simulink model "pv_model"  (R2020a)
settings: Solver=VariableStepAuto  StartTime=0.0  StopTime=4  RelTol=1e-3
undefined symbols (not defined in the file): Eg0, Isc, K, Ki, n, Ns, q, Rs, Rsh, Tn, Voc
libraries: simulink x3
settings Model: Creator=vardh  LastModifiedBy=vardh
settings SolverCC: AlgebraicLoopSolver=LineSearch
settings DebuggingCC: AlgebraicLoopMsg=none

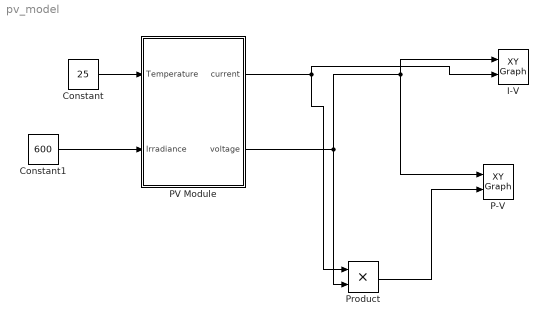
== system pv_model ==
  Constant : Constant  Value=25
  Constant1 : Constant  Value=600
  "I-V " : simulink/Sinks/XY Graph  xmin=0  xmax=35  ymin=0  ymax=10  st=-1
  P-V : simulink/Sinks/XY Graph  xmin=0  xmax=35  ymin=0  ymax=210  st=-1
  PV Module : Subsystem  InitFcn=|
      | Ki=0.0032;
      | q=1.6e-19;
      | K=1.38e-23;
      | n=1.3;
      | Eg0=1.1;
      | Rs=0.221;
      | Rsh=415.405;
      | Tn=298;
      | Voc=32.9;
      | Isc=8.21;
      | Ns=54;
  Product : Product
  wires:
  Constant/1 -> PV Module/1(Temperature)
  Constant1/1 -> PV Module/2(Irradiance)
  PV Module/1(current) -> Product/1, "I-V "/2
  PV Module/2(voltage) -> P-V/1, "I-V "/1, Product/2
  Product/1 -> P-V/2

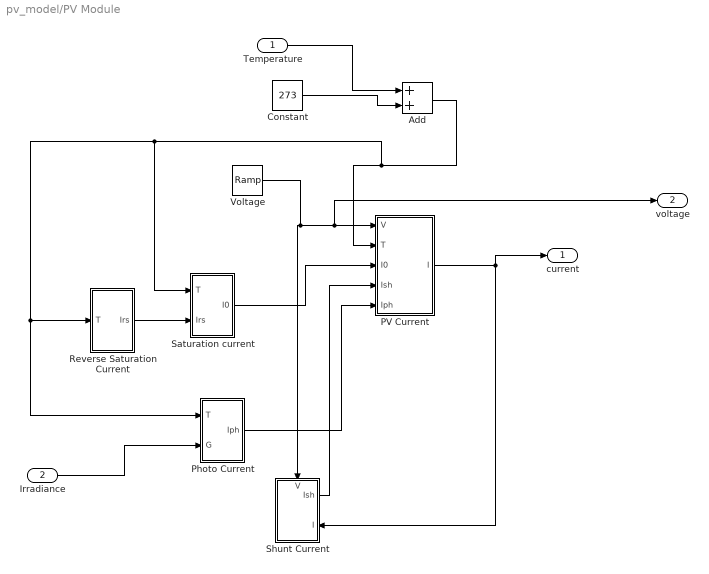
== system pv_model/PV Module ==
  Temperature : Inport
  Irradiance : Inport  Port=2
  Add : Sum
  Constant : Constant  Value=273
  PV Current : Subsystem
  Photo Current : Subsystem
  Reverse Saturation Current : Subsystem
  Saturation current : Subsystem
  Shunt Current : Subsystem
      settings: PortSchema="{\"entries\":[{\"content\":{\"sides\":[{\"content\":{\"connectorIds\":[]},\"type\":\"ConnectorPlacement.EquallySpacedRectSide\",\"uuid\":\"dfbb4c5d-8fcf-4819-9965-5f47220c7753\"},{\"content\":{\"connectorIds\":[\"Out1\",\"In2\"],\"side\":\"RIGHT\"},\"type\":\"ConnectorPlacement.EquallySpacedRectSide\",\"uuid\":\"987aa4c6-8b7c-4032-9cd9-5753be429a4d\"},{\"content\":{\"connectorIds\":[\"In1\"],\"side\":\"TOP\"},\"type\":\"ConnectorPlacement.EquallySpacedRectSide\",\"uuid\":\"a02384b8-48a1-4401-ad36-e6b05eaf9311\"}]},\"type\":\"ConnectorPlacement.EquallySpacedConnector\",\"uuid\":\"4fb9e7c8-c8f8-43f6-a1be-daa0a140ff41\"}],\"packageUris\":[\"http://schema.mathworks.com/mf0/Connector/19700101\"],\"version\":\"1.0\"}"
  Voltage : simulink/Sources/Ramp  slope=10  start=0  InitialOutput=0
  current : Outport
  voltage : Outport  Port=2
  wires:
  Voltage/1 -> voltage/1, PV Current/1(V), Shunt Current/1(V)
  Irradiance/1 -> Photo Current/2(G)
  Constant/1 -> Add/2
  Add/1 -> Saturation current/1(T), Reverse Saturation Current/1(T), Photo Current/1(T), PV Current/2(T)
  PV Current/1(I) -> current/1, Shunt Current/2(I)
  Saturation current/1(I0) -> PV Current/3(I0)
  Temperature/1 -> Add/1
  Reverse Saturation Current/1(Irs) -> Saturation current/2(Irs)
  Photo Current/1(Iph) -> PV Current/5(Iph)
  Shunt Current/1(Ish) -> PV Current/4(Ish)

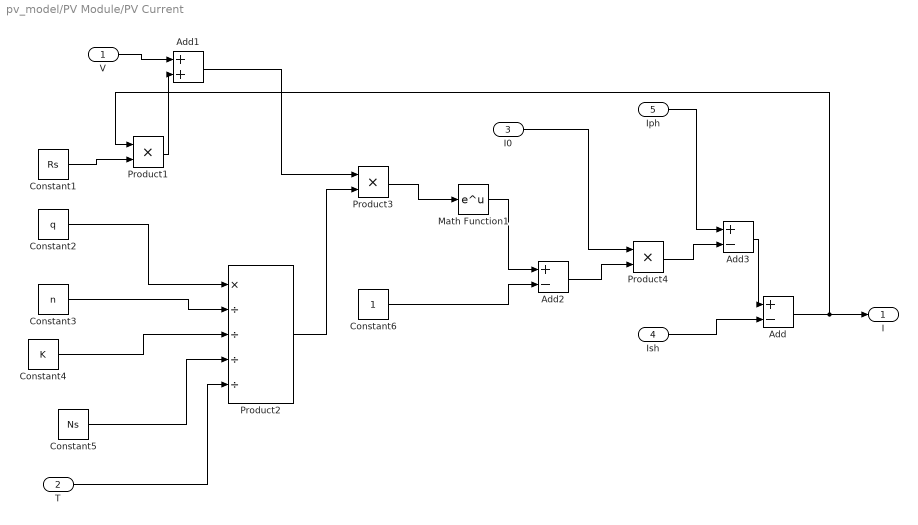
== system pv_model/PV Module/PV Current ==
  V : Inport
  T : Inport  Port=2
  I0 : Inport  Port=3
  Ish : Inport  Port=4
  Iph : Inport  Port=5
  Add : Sum  Inputs=+-
  Add1 : Sum
  Add2 : Sum  Inputs=+-
  Add3 : Sum  Inputs=+-
  Constant1 : Constant  Value=Rs
  Constant2 : Constant  Value=q
  Constant3 : Constant  Value=n
  Constant4 : Constant  Value=K
  Constant5 : Constant  Value=Ns
  Constant6 : Constant
  Math Function1 : Math  SaturateOnIntegerOverflow=on
  Product1 : Product
  Product2 : Product  Inputs=*////
  Product3 : Product
  Product4 : Product
  I : Outport
  wires:
  Product3/1 -> Math Function1/1
  Constant1/1 -> Product1/2
  Add3/1 -> Add/1
  T/1 -> Product2/5
  Constant5/1 -> Product2/4
  Constant2/1 -> Product2/1
  Add2/1 -> Product4/2
  Constant3/1 -> Product2/2
  Constant4/1 -> Product2/3
  Product2/1 -> Product3/2
  Iph/1 -> Add3/1
  Math Function1/1 -> Add2/1
  Product4/1 -> Add3/2
  V/1 -> Add1/1
  Add/1 -> I/1, Product1/1
  Constant6/1 -> Add2/2
  Product1/1 -> Add1/2
  I0/1 -> Product4/1
  Add1/1 -> Product3/1
  Ish/1 -> Add/2

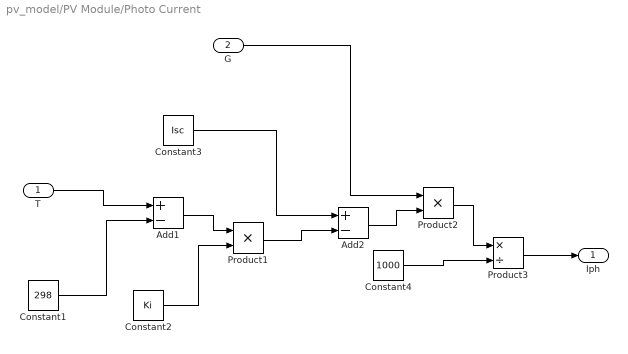
== system pv_model/PV Module/Photo Current ==
  T : Inport
  G : Inport  Port=2
  Add1 : Sum  Inputs=+-
  Add2 : Sum  Inputs=+-
  Constant1 : Constant  Value=298
  Constant2 : Constant  Value=Ki
  Constant3 : Constant  Value=Isc
  Constant4 : Constant  Value=1000
  Product1 : Product
  Product2 : Product
  Product3 : Product  Inputs=*/
  Iph : Outport
  wires:
  Add2/1 -> Product2/2
  Constant3/1 -> Add2/1
  Constant4/1 -> Product3/2
  Product3/1 -> Iph/1
  Product1/1 -> Add2/2
  Add1/1 -> Product1/1
  G/1 -> Product2/1
  Product2/1 -> Product3/1
  Constant1/1 -> Add1/2
  T/1 -> Add1/1
  Constant2/1 -> Product1/2

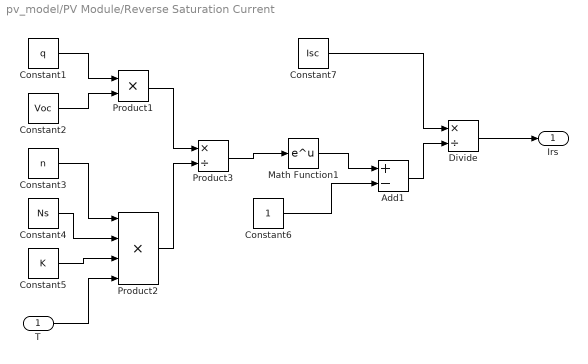
== system pv_model/PV Module/Reverse Saturation Current ==
  T : Inport
  Add1 : Sum  Inputs=+-
  Constant1 : Constant  Value=q
  Constant2 : Constant  Value=Voc
  Constant3 : Constant  Value=n
  Constant4 : Constant  Value=Ns
  Constant5 : Constant  Value=K
  Constant6 : Constant
  Constant7 : Constant  Value=Isc
  Divide : Product  Inputs=*/
  Math Function1 : Math  SaturateOnIntegerOverflow=on
  Product1 : Product
  Product2 : Product  Inputs=4
  Product3 : Product  Inputs=*/
  Irs : Outport
  wires:
  Product2/1 -> Product3/2
  Constant3/1 -> Product2/1
  Constant6/1 -> Add1/2
  Constant4/1 -> Product2/2
  Constant2/1 -> Product1/2
  Product1/1 -> Product3/1
  Constant5/1 -> Product2/3
  Math Function1/1 -> Add1/1
  Constant1/1 -> Product1/1
  Divide/1 -> Irs/1
  Product3/1 -> Math Function1/1
  T/1 -> Product2/4
  Add1/1 -> Divide/2
  Constant7/1 -> Divide/1

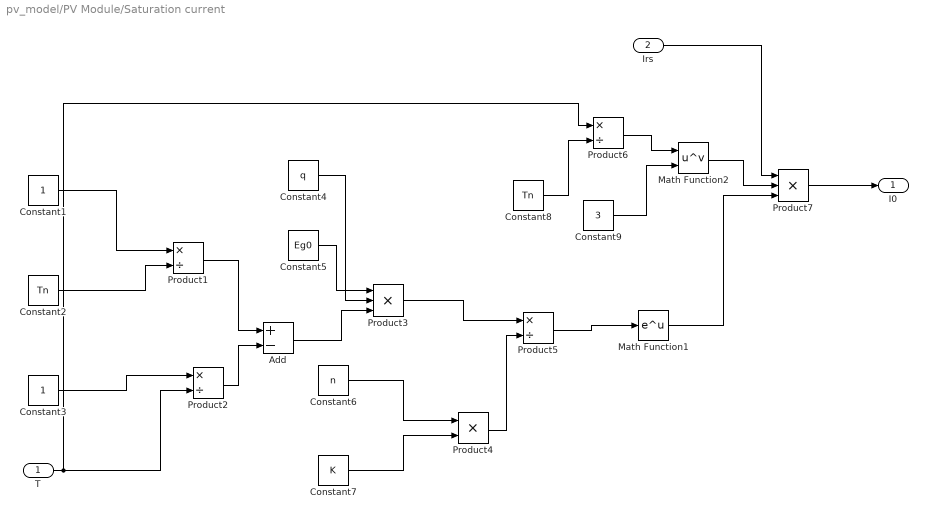
== system pv_model/PV Module/Saturation current ==
  T : Inport
  Irs : Inport  Port=2
  Add : Sum  Inputs=+-
  Constant1 : Constant
  Constant2 : Constant  Value=Tn
  Constant3 : Constant
  Constant4 : Constant  Value=q
  Constant5 : Constant  Value=Eg0
  Constant6 : Constant  Value=n
  Constant7 : Constant  Value=K
  Constant8 : Constant  Value=Tn
  Constant9 : Constant  Value=3
  Math Function1 : Math  SaturateOnIntegerOverflow=on
  Math Function2 : Math  Operator=pow  SaturateOnIntegerOverflow=on
  Product{1..2,5..6} (4 alike) : Product  Inputs=*/
  Product3 : Product  Inputs=***
  Product4 : Product
  Product7 : Product  Inputs=3
  I0 : Outport
  wires:
  Product7/1 -> I0/1
  Constant1/1 -> Product1/1
  Constant2/1 -> Product1/2
  Product4/1 -> Product5/2
  Constant9/1 -> Math Function2/2
  Product3/1 -> Product5/1
  Constant6/1 -> Product4/1
  Add/1 -> Product3/3
  Irs/1 -> Product7/1
  T/1 -> Product2/2, Product6/1
  Math Function2/1 -> Product7/2
  Constant5/1 -> Product3/1
  Math Function1/1 -> Product7/3
  Constant8/1 -> Product6/2
  Product6/1 -> Math Function2/1
  Product1/1 -> Add/1
  Product5/1 -> Math Function1/1
  Constant3/1 -> Product2/1
  Product2/1 -> Add/2
  Constant4/1 -> Product3/2
  Constant7/1 -> Product4/2

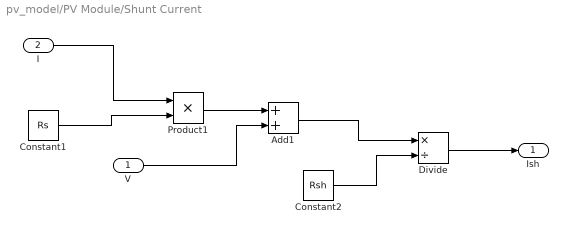
== system pv_model/PV Module/Shunt Current ==
  V : Inport
  I : Inport  Port=2
  Add1 : Sum
  Constant1 : Constant  Value=Rs
  Constant2 : Constant  Value=Rsh
  Divide : Product  Inputs=*/
  Product1 : Product
  Ish : Outport
  wires:
  Add1/1 -> Divide/1
  Product1/1 -> Add1/1
  I/1 -> Product1/1
  Constant2/1 -> Divide/2
  Constant1/1 -> Product1/2
  Divide/1 -> Ish/1
  V/1 -> Add1/2
